simulink model "Problem5"  (R2020a)
settings: Solver=VariableStepAuto  StartTime=0.0  StopTime=10.0  RelTol=1e-3
model workspace (MAT data in the model file):
  C = 1e-05
  R = 10
  q = 5
settings Model: Creator=sreeram  LastModifiedBy=sreeram

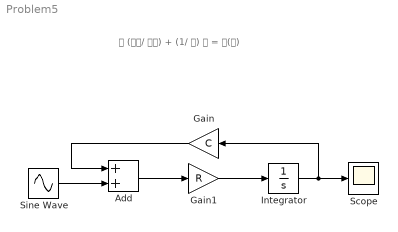
== system Problem5 ==
  note: 𝑅 (𝑑𝑄/ 𝑑𝑡) + (1/ 𝐶) 𝑄 = 𝐸(𝑡)
  Add : Sum
  Gain : Gain  Gain=C
  Gain1 : Gain  Gain=R
  Integrator : Integrator
  Scope : Scope
  Sine Wave : Sin  Amplitude=10  Frequency=2*pi*200  SampleTime=0
  wires:
  Sine Wave/1 -> Add/2
  Gain/1 -> Add/1
  Add/1 -> Gain1/1
  Gain1/1 -> Integrator/1
  Integrator/1 -> Gain/1, Scope/1
